simulink model "motorcontrol_codegen_19a"  (R2019a)
settings: Solver=FixedStepDiscrete  StartTime=0.0  StopTime=Inf  MaxStep=5e-5  RelTol=1e-3  EnableMultiTasking=on
values from neighbouring files (symbols this model uses):
  dataType = 'single'    [motorcontrol_codegen_params.m]
undefined symbols (not defined in the file or in its folder): ControlMode, ctrlParams, DiscIntNeverNeededParam, Down, GPTRIP1SEL, GPTRIP2SEL, inverter, mcb_isSimVar, NumBits1, NumBits2, PI_params, pmsm, Slope1, Slope2, Target, Ts, TZ1, TZ2, Up
libraries: simulink x14, c2802xlib x5, c2837xDlib x4, c280xlib x1, c2000lib x1
(part 3 of 3)

== system motorcontrol_codegen_19a/Motor_Control1/ControlSystem/Open Loop Start-Up/Subsystem1/Subsystem1 ==
  In1 : Inport
  In2 : Inport  Port=2
  Data Type Duplicate : DataTypeDuplicate
  add_b : Sum  Inputs=-+  RndMeth=Simplest  OutDataTypeStr=Inherit: Same as first input
  add_c : Sum  Inputs=--  RndMeth=Simplest  OutDataTypeStr=Inherit: Same as first input
  one_by_two : Gain  Gain=1/2  RndMeth=Simplest  OutDataTypeStr=Inherit: Same as input
  sqrt3_by_two : Gain  Gain=sqrt(3)/2  RndMeth=Simplest  OutDataTypeStr=Inherit: Same as input
  a : Outport  VectorParamsAs1DForOutWhenUnconnected=off
  b : Outport  Port=2  VectorParamsAs1DForOutWhenUnconnected=off
  c : Outport  Port=3  VectorParamsAs1DForOutWhenUnconnected=off
  wires:
  add_c/1 -> c/1
  one_by_two/1 -> add_b/1, add_c/1
  In2/1 -> sqrt3_by_two/1, Data Type Duplicate/2
  sqrt3_by_two/1 -> add_c/2, add_b/2
  add_b/1 -> b/1
  In1/1 -> one_by_two/1, Data Type Duplicate/1, a/1

== system motorcontrol_codegen_19a/Motor_Control1/ControlSystem/Open Loop Start-Up/Subsystem1/Subsystem2 ==
  Ds : Inport
  Qs : Inport  Port=2
  sin : Inport  Port=3
  cos : Inport  Port=4
  Data Type Duplicate : DataTypeDuplicate  NumInputPorts=4
  Subsystem : Subsystem
  dcos : Product  RndMeth=Simplest  OutDataTypeStr=Inherit: Same as first input
  dsin : Product  RndMeth=Simplest  OutDataTypeStr=Inherit: Same as first input
  qcos : Product  RndMeth=Simplest  OutDataTypeStr=Inherit: Same as first input
  qsin : Product  RndMeth=Simplest  OutDataTypeStr=Inherit: Same as first input
  sum_alpha : Sum  Inputs=|+-  RndMeth=Simplest  OutDataTypeStr=Inherit: Same as first input
  sum_beta : Sum  Inputs=|++  RndMeth=Simplest  OutDataTypeStr=Inherit: Same as first input
  Alpha : Outport  VectorParamsAs1DForOutWhenUnconnected=off
  Beta : Outport  Port=2  VectorParamsAs1DForOutWhenUnconnected=off
  wires:
  cos/1 -> qcos/2, dcos/2, Data Type Duplicate/3
  qsin/1 -> sum_alpha/2
  Subsystem/1(Alpha) -> Alpha/1
  Qs/1 -> qsin/1, qcos/1, Data Type Duplicate/2
  sum_beta/1 -> Subsystem/2(B)
  qcos/1 -> sum_beta/1
  dcos/1 -> sum_alpha/1
  Ds/1 -> dcos/1, dsin/1, Data Type Duplicate/1
  Subsystem/2(Beta) -> Beta/1
  sin/1 -> dsin/2, qsin/2, Data Type Duplicate/4
  sum_alpha/1 -> Subsystem/1(A)
  dsin/1 -> sum_beta/2

== system motorcontrol_codegen_19a/Motor_Control1/Input Scaling/ Calculate Position and Speed/Subsystem2/PositionNoReset ==
  Index : Inport
  Count : Inport  Port=2
  Action Port : ActionPort
  CountsPerRevolution : Constant  Value=EncoderSlitsPerRevolution*4  OutDataTypeStr=Inherit: Inherit via back propagation
  MinMax : MinMax  Inputs=2  RndMeth=Simplest  ZeroCross=off
  Sum3 : Sum  Inputs=+-|  OutDataTypeStr=Inherit: Same as accumulator  RndMeth=Simplest
  Sum7 : Sum  Inputs=|++  OutDataTypeStr=Inherit: Same as accumulator  RndMeth=Simplest
  Position : Outport  VectorParamsAs1DForOutWhenUnconnected=off
  wires:
  Sum3/1 -> MinMax/1, Sum7/1
  Count/1 -> Sum3/1
  Index/1 -> Sum3/2
  CountsPerRevolution/1 -> Sum7/2
  Sum7/1 -> MinMax/2
  MinMax/1 -> Position/1

== system motorcontrol_codegen_19a/Motor_Control1/Input Scaling/ Calculate Position and Speed/Subsystem2/PositionResetatIndex ==
  Count : Inport
  Action Port : ActionPort
  Position : Outport  VectorParamsAs1DForOutWhenUnconnected=off
  wires:
  Count/1 -> Position/1

== system motorcontrol_codegen_19a/Motor_Control1/Input Scaling/ Calculate Position and Speed/Subsystem3/Subsystem ==
  ϴm : Inport
  In2 : Inport  Port=2
  If : If  NumInputs=2  IfExpression=u1 <= u2
  Merge : Merge
  Subsystem : Subsystem
  Subsystem1 : Subsystem
  Out1 : Outport
  wires:
  Merge/1 -> Out1/1
  If/2 -> Subsystem1/Action
  Subsystem/1(Out1) -> Merge/1
  ϴm/1 -> If/1, Subsystem/1(ϴm), Subsystem1/1(ϴm)
  If/1 -> Subsystem/Action
  Subsystem1/1(Out1) -> Merge/2
  In2/1 -> Subsystem/2(In2), Subsystem1/2(In2), If/2

== system motorcontrol_codegen_19a/Motor_Control1/Input Scaling/ Calculate Position and Speed/Subsystem3/Subsystem1 ==
  In1 : Inport
  Add : Sum  Inputs=-+  OutDataTypeStr=Inherit: Inherit via back propagation  RndMeth=Simplest
  Floor : Rounding
  Multiply : Gain  Gain=1/maxAngleIn  RndMeth=Simplest  OutDataTypeStr=Inherit: Same as input
  Multiply1 : Gain  Gain=maxAngleIn  OutDataTypeStr=Inherit: Inherit via back propagation  RndMeth=Simplest
  Number of pole pairs : Gain  Gain=NrPP  RndMeth=Simplest  OutDataTypeStr=Inherit: Same as input
  Out1 : Outport
  ϴe : Outport  Port=2
  wires:
  Multiply1/1 -> Add/1
  Number of pole pairs/1 -> Multiply/1, Add/2
  Add/1 -> ϴe/1, Out1/1
  Floor/1 -> Multiply1/1
  Multiply/1 -> Floor/1
  In1/1 -> Number of pole pairs/1

== system motorcontrol_codegen_19a/Motor_Control1/ControlSystem/Closed_Loop/Sine-Cosine Lookup/Subsystem/Subsystem ==
  In1 : Inport
  Action Port : ActionPort
  Convert_back : DataTypeConversion  RndMeth=Simplest
  Convert_uint16 : DataTypeConversion  OutDataTypeStr=int16
  Data Type Duplicate : DataTypeDuplicate
  Sum : Sum  Inputs=|+-  RndMeth=Simplest  OutDataTypeStr=Inherit: Same as first input
  Out1 : Outport
  wires:
  In1/1 -> Data Type Duplicate/1, Sum/1, Convert_uint16/1
  Convert_uint16/1 -> Convert_back/1
  Convert_back/1 -> Sum/2, Data Type Duplicate/2
  Sum/1 -> Out1/1

== system motorcontrol_codegen_19a/Motor_Control1/ControlSystem/Closed_Loop/Sine-Cosine Lookup/Subsystem/Subsystem1 ==
  In1 : Inport
  Action Port : ActionPort
  Convert_back : DataTypeConversion  RndMeth=Simplest
  Convert_uint16 : DataTypeConversion  OutDataTypeStr=int16  RndMeth=Simplest
  Data Type Duplicate : DataTypeDuplicate
  Sum : Sum  Inputs=|+-  RndMeth=Simplest  OutDataTypeStr=Inherit: Same as first input
  Out1 : Outport
  wires:
  Convert_uint16/1 -> Convert_back/1
  In1/1 -> Data Type Duplicate/1, Sum/1, Convert_uint16/1
  Convert_back/1 -> Sum/2, Data Type Duplicate/2
  Sum/1 -> Out1/1

== system motorcontrol_codegen_19a/Motor_Control1/ControlSystem/Open Loop Start-Up/Subsystem1/Sine-Cosine Lookup/Subsystem ==
  In1 : Inport
  Compare To Zero : simulink/Logic and Bit Operations/Compare To Zero  relop=<  OutDataTypeStr=boolean
  Data Type Conversion : DataTypeConversion  OutDataTypeStr=uint16  ConvertRealWorld=Stored Integer (SI)  RndMeth=Simplest
  If : If
  Merge : Merge
  Subsystem : Subsystem
  Subsystem1 : Subsystem
  convert_pu : Gain  Gain=1/(dlgSett.UpperSatLimit)  RndMeth=Simplest  OutDataTypeStr=Inherit: Same as input
  Out1 : Outport
  wires:
  If/2 -> Subsystem1/Action
  Subsystem/1(Out1) -> Merge/1
  convert_pu/1 -> Subsystem1/1(In1), Subsystem/1(In1), Compare To Zero/1
  In1/1 -> convert_pu/1
  If/1 -> Subsystem/Action
  Subsystem1/1(Out1) -> Merge/2
  Data Type Conversion/1 -> If/1
  Compare To Zero/1 -> Data Type Conversion/1
  Merge/1 -> Out1/1

== system motorcontrol_codegen_19a/Motor_Control1/ControlSystem/Open Loop Start-Up/Subsystem1/Sine-Cosine Lookup/Subsystem1 ==
  In1 : Inport
  In2 : Inport  Port=2
  Demux : Demux
  Product : Product  RndMeth=Simplest  OutDataTypeStr=Inherit: Same as first input
  Product1 : Product  RndMeth=Simplest  OutDataTypeStr=Inherit: Same as first input
  Sum3 : Sum  Inputs=|+-  RndMeth=Simplest  OutDataTypeStr=Inherit: Same as first input
  Sum4 : Sum  Inputs=|++  RndMeth=Simplest  OutDataTypeStr=Inherit: Same as first input
  Sum5 : Sum  Inputs=|+-  RndMeth=Simplest  OutDataTypeStr=Inherit: Same as first input
  Sum6 : Sum  Inputs=|++  RndMeth=Simplest  OutDataTypeStr=Inherit: Same as first input
  Out1 : Outport
  Out2 : Outport  Port=2
  wires:
  Sum4/1 -> Out1/1
  Sum5/1 -> Product1/1
  Sum6/1 -> Out2/1
  Demux/1 -> Sum3/1
  Demux/2 -> Sum4/2, Sum3/2
  Product/1 -> Sum4/1
  Sum3/1 -> Product/1
  Product1/1 -> Sum6/1
  Demux/4 -> Sum5/2, Sum6/2
  In1/1 -> Demux/1
  Demux/3 -> Sum5/1
  In2/1 -> Product1/2, Product/2

== system motorcontrol_codegen_19a/Motor_Control1/ControlSystem/Open Loop Start-Up/Subsystem1/Subsystem2/Subsystem ==
  A : Inport
  B : Inport  Port=2
  D_axis_aligned : Mux  Inputs=2
  Demux : Demux  Outputs=2
  Offset : Constant  Value=dlgSett.Offset  OutDataTypeStr=uint16  SampleTime=-1
  Q_axis_aligned : Mux  Inputs=2
  Switch : Switch  Criteria=u2 > Threshold  Threshold=1  RndMeth=Simplest  ZeroCross=off
  Unary_Minus : UnaryMinus
  Alpha : Outport  VectorParamsAs1DForOutWhenUnconnected=off
  Beta : Outport  Port=2  VectorParamsAs1DForOutWhenUnconnected=off
  wires:
  Unary_Minus/1 -> Q_axis_aligned/2
  Offset/1 -> Switch/2
  B/1 -> D_axis_aligned/2, Q_axis_aligned/1
  Demux/2 -> Beta/1
  A/1 -> D_axis_aligned/1, Unary_Minus/1
  Switch/1 -> Demux/1
  D_axis_aligned/1 -> Switch/3
  Demux/1 -> Alpha/1
  Q_axis_aligned/1 -> Switch/1

== system motorcontrol_codegen_19a/Motor_Control1/Input Scaling/ Calculate Position and Speed/Subsystem3/Subsystem/Subsystem ==
  ϴm : Inport
  In2 : Inport  Port=2
  Action Port : ActionPort
  Add : Sum  Inputs=++-  RndMeth=Simplest  OutDataTypeStr=Inherit: Same as first input
  Constant : Constant  Value=maxAngleIn  OutDataTypeStr=Inherit: Inherit via back propagation
  Out1 : Outport
  wires:
  Add/1 -> Out1/1
  ϴm/1 -> Add/1
  Constant/1 -> Add/2
  In2/1 -> Add/3

== system motorcontrol_codegen_19a/Motor_Control1/Input Scaling/ Calculate Position and Speed/Subsystem3/Subsystem/Subsystem1 ==
  ϴm : Inport
  In2 : Inport  Port=2
  Action Port : ActionPort
  Add : Sum  Inputs=+-  RndMeth=Simplest  OutDataTypeStr=Inherit: Same as first input
  Out1 : Outport
  wires:
  Add/1 -> Out1/1
  ϴm/1 -> Add/1
  In2/1 -> Add/2

== system motorcontrol_codegen_19a/Motor_Control1/ControlSystem/Open Loop Start-Up/Subsystem1/Sine-Cosine Lookup/Subsystem/Subsystem ==
  In1 : Inport
  Action Port : ActionPort
  Convert_back : DataTypeConversion  RndMeth=Simplest
  Convert_uint16 : DataTypeConversion  OutDataTypeStr=int16
  Data Type Duplicate : DataTypeDuplicate
  Sum : Sum  Inputs=|+-  RndMeth=Simplest  OutDataTypeStr=Inherit: Same as first input
  Out1 : Outport
  wires:
  In1/1 -> Data Type Duplicate/1, Sum/1, Convert_uint16/1
  Convert_uint16/1 -> Convert_back/1
  Convert_back/1 -> Sum/2, Data Type Duplicate/2
  Sum/1 -> Out1/1

== system motorcontrol_codegen_19a/Motor_Control1/ControlSystem/Open Loop Start-Up/Subsystem1/Sine-Cosine Lookup/Subsystem/Subsystem1 ==
  In1 : Inport
  Action Port : ActionPort
  Convert_back : DataTypeConversion  RndMeth=Simplest
  Convert_uint16 : DataTypeConversion  OutDataTypeStr=int16  RndMeth=Simplest
  Data Type Duplicate : DataTypeDuplicate
  Sum : Sum  Inputs=|+-  RndMeth=Simplest  OutDataTypeStr=Inherit: Same as first input
  Out1 : Outport
  wires:
  Convert_uint16/1 -> Convert_back/1
  In1/1 -> Data Type Duplicate/1, Sum/1, Convert_uint16/1
  Convert_back/1 -> Sum/2, Data Type Duplicate/2
  Sum/1 -> Out1/1

== stateflow chart motorcontrol_codegen_19a/Mode_Scheduler/Controller_Mode_Scheduler ==
  settings: updateMethod=DISCRETE  executeAtInitialization=1
  note: Controller Mode Scheduler
  note: The motor control algorithm begins in a stand-by mode awaiting a command to turn the motor on. Once this command
      | is issued the motor rotates to identify a known rotor position with valid position. The appropriate closed loop control then begins.
      | Upon a request to stop the motor, the motor will decellerate until zero speed is identified, after which the algorithm returns to the stand-by mode.
  state Stand_By
    entry: controller_mode = SpeedControl;
    velocity_command=0;
    torque_command = 0;
  state Motor_On
    state Motor_Control
      state Speed_Control
        entry: controller_mode = SpeedControl;
        en, du:
        velocity_command = command;
      state Position_Control
        entry: controller_mode = PositionControl;
        en,du:
        position_command = command;
      state Torque_Control
        entry: controller_mode = TorqueControl;
        en, du:
        torque_command = command;
      (default) -> (junction 386)
      (junction 386) -> Speed_Control [order 1] : [command_type==Speed]
      (junction 386) -> (junction 387) [order 2]
      (junction 387) -> Position_Control [order 1] : [command_type==Position]
      (junction 387) -> (junction 388) [order 2]
      (junction 388) -> Torque_Control : % [command_type==Torque]
  (default) -> Stand_By
  Stand_By -> Motor_On : [motor_on]
  Motor_On -> Stand_By : [~motor_on]
  data: controller_mode output Enum: ControllerMode; velocity_command output dataType; motor_on input boolean; position_command output dataType; command_type input Enum: ControlMode; torque_command output dataType; command input dataType
